simulink model "FlashMemory"  (R2016b)
settings: Solver=FixedStepAuto  StartTime=0.0  StopTime=10.0  RelTol=1e-3
PreLoadFcn:
  | waijung.modelPreload; % Required for working with Waijung Blockset. Do not remove.
undefined symbols (not defined in the file): CPHA_1Edge, CPOL_Low, deg_, Duplex, FirstBit_MSB, Full, g, imu, Link, LQFP100, ST, STM32F407VG, STM32F4DISCOVERY, Ts
libraries: simulink x45, stm32f4_i2c_lib x12, stm32f4_spi_lib x4, stm32f4_flash_lib x3, stm32f4_io_lib x1, cube_lib x1, stm32f4_device_config_lib x1, BC_USB x1
(part 1 of 3)
CloseFcn:
  | waijung.modelClose; % Required for working with Waijung Blockset. Do not remove.
settings Model: Creator=Wall  LastModifiedBy=Wall
settings OptimizationCC: DefaultParameterBehavior=Inlined
settings DebuggingCC: ParameterTunabilityLossMsg=error
settings HardwareCC: ProdBitPerPointer=32  ProdBitPerSizeT=32  ProdBitPerPtrDiffT=32  ProdLargestAtomicFloat=None  ProdIntDivRoundTo=Undefined  ProdWordSize=32  ProdHWDeviceType=ARM Compatible->Cortex - M4  TargetEndianess=LittleEndian  TargetHWDeviceType=ARM Compatible->Cortex - M4
settings RTWCC: SystemTargetFile=stm32f4.tlc  GenerateMakefile=off  TemplateMakefile=ert_default_tmf  Description=STM32F4 Target  GenerateReport=on  IncludeHyperlinkInReport=on  GenerateTraceInfo=on  GenerateTraceReport=on  GenerateTraceReportSl=on  GenerateTraceReportSf=on  GenerateTraceReportEml=on
settings CodeAppCC: ForceParamTrailComments=on  IgnoreCustomStorageClasses=off  OperatorAnnotations=on  SimulinkDataObjDesc=on  SFDataObjDesc=on  MATLABFcnDesc=on  InsertBlockDesc=on  MATLABSourceComments=on
settings STFCustomTargetCC: TargetLangStandard=C99 (ISO)  ModelReferenceCompliant=off  CombineOutputUpdateFcns=on  ERTCustomFileBanners=on  SupportContinuousTime=off  SupportNonInlinedSFcns=off  RemoveResetFunc=on  MATLABClassNameForMDSCustomization=Simulink.SoftwareTarget.ERTCustomization  GRTInterface=off  SystemTargetFile=stm32f4.tlc
settings ERTTargetCC: TargetLangStandard=C99 (ISO)  ModelReferenceCompliant=off  ParMdlRefBuildCompliant=off  CompOptLevelCompliant=off  ConcurrentExecutionCompliant=off  ERTFirstTimeCompliant=off  ModelStepFunctionPrototypeControlCompliant=off  CPPClassGenCompliant=off  UseToolchainInfoCompliant=off  InlinedParameterPlacement=NonHierarchical  ERTSrcFileBannerTemplate=stm32f4_code_template.cgt  ERTHdrFileBannerTemplate=stm32f4_code_template.cgt  ERTDataSrcFileTemplate=stm32f4_code_template.cgt  ERTDataHdrFileTemplate=stm32f4_code_template.cgt  ERTCustomFileTemplate=stm32f4_file_process.tlc

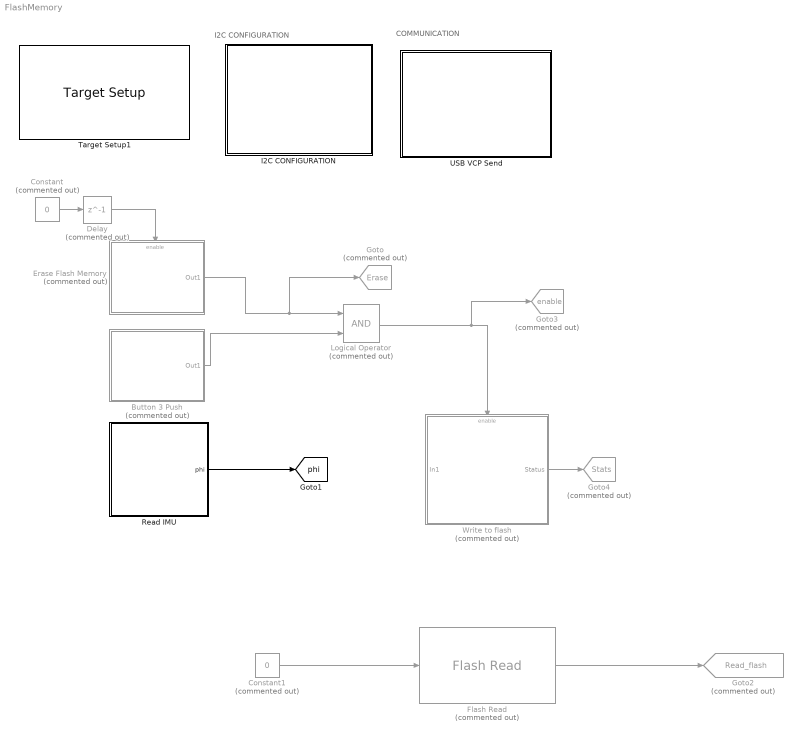
== system FlashMemory ==
  note: COMMUNICATION
  note: I2C CONFIGURATION
  Button 3 Push : Subsystem  Commented=on
  Constant : Constant  Commented=on  Value=0  SampleTime=Ts.IMU
  Constant1 : Constant  Commented=on  Value=0  OutDataTypeStr=uint32  SampleTime=-1
  Delay : Delay  Commented=on  DelayLength=1  InitialCondition=1
  Erase Flash Memory : Subsystem  Commented=on
  Flash Read : stm32f4_flash_lib/Flash Read  Commented=on  conf=Read  transfer=Blocking  flashsector=Sector 6: 0x08040000 - 0x0805FFFF  datatype=single  datacount=1  enablestatus=on  sampletime=Ts.IMU  sampletimestr=0.008  blockid=FlashRead  inputarray=[-1]  inputlabelarray={'Offset '}  outputarray=[1]  outputlabelarray={'Data (single)'}  compat=0  confstr="[\"single\",\"20000\",\"08040000\",\"6\",\"on\"]"
  Goto : Goto  Commented=on  GotoTag=Erase  TagVisibility=global
  Goto2 : Goto  Commented=on  GotoTag=Read_flash  TagVisibility=global
  Goto3 : Goto  Commented=on  GotoTag=enable  TagVisibility=global
  Goto4 : Goto  Commented=on  GotoTag=Stats  TagVisibility=global
  I2C CONFIGURATION : Subsystem
  Logical Operator : Logic  Commented=on  AllPortsSameDT=off  OutDataTypeStr=boolean
  Read IMU : Subsystem
  Target Setup1 : stm32f4_device_config_lib/Target Setup  Priority=100  compiler=GNU ARM  previous_compiler=GNU ARM  mcu=STM32F407VG (LQFP100); STM32F4DISCOVERY  mcustr=STM32F407VG  clockconfig=STM32F4DISCOVERY Default (HSEOSC-8MHz/HCLK-168MHz)  system_stm32f4xx_c_path=C:\waijung15_04a\targets\stm32f4_target\stm32f4\utils\STM32F4xx_AN3988_V1.0.1\stm32f4_default\hseosc8mhz  showmemoryconfiguration=off  stacksize=0x400  heapsize=0x200  enableautocompiledownload=on  fullchiperase=off  programmerinterface=ST-Link  editctrlstr=on  compilercontrolstr=$(patsubst %, -I%, .) -mcpu=cortex-m4 -mthumb -mthumb-interwork -mfloat-abi=hard -mfpu=fpv4-sp-d16 -ffast-math -Wall -Wextra -Ofast  assemblercontrolstr=$(patsubst %, -I%, .) -mcpu=cortex-m4 -mthumb -mthumb-interwork -mfloat-abi=hard -mfpu=fpv4-sp-d16 -ffast-math -Wall -Wextra -Ofast -Wa,-amhls=$(<:.s=.lst) -D__STACK_SIZE=$(STACK_SIZE) -D__HEAP_SIZE=$(HEAP_SIZE)  linkercontrolstr=-T$(LD_SCRIPT) -g -Wl,-Map=$(MAP),--cref,--no-warn-mismatch -mcpu=cortex-m4 -mthumb -mthumb-interwork -mfloat-abi=hard -mfpu=fpv4-sp-d16  runafterdownload=on  execprofile=None  profileruart=1  profilerbaud=115200  profilertxpin=Not used  profilerinitstr=0.002,168000000,336000,115200,0  manualsetsampletime=on  sampletime=0.002  blockid=TargetSetup1  systickreloadvalue=336000  hseval=8000000  lastprofileruart=1  hclk=168000000  flashorigin=0x8000000  flashlength=1M  ramorigin=0x20000000  ramlength=112k  useextram=off
  USB VCP Send : Subsystem
  Write to flash : Subsystem  Commented=on
  tag scope: phi=global
  wires:
  Constant/1 -> Delay/1
  Delay/1 -> Erase Flash Memory/Enable
  Erase Flash Memory/1(Out1) -> Goto/1, Logical Operator/1
  Logical Operator/1 -> Goto3/1, Write to flash/Enable
  Button 3 Push/1(Out1) -> Logical Operator/2
  Read IMU/1(phi) -> [phi]
  Constant1/1 -> Flash Read/1
  Write to flash/1(Status) -> Goto4/1
  Flash Read/1 -> Goto2/1

== system FlashMemory/Button 3 Push ==
  Buttom 3 : stm32f4_io_lib/Digital Input  port=E  speed=100  porttype=Pull Up  porttypestr=UP  use_pin0=off  use_pin1=off  use_pin2=off  use_pin3=off  use_pin4=off  use_pin5=off  use_pin6=off  use_pin7=off  use_pin8=off  use_pin9=off  use_pin10=on  use_pin11=off  use_pin12=off  use_pin13=off  use_pin14=off  use_pin15=off  pinstr=GPIO_Pin_10  usedpinarray="[0  0  0  0  0  0  0  0  0  0  1  0  0  0  0  0]"  bitbandingstr="#define Button3PushButtom3_E10 Peripheral_BB(GPIOE->IDR, 10)  /* Output pin */"  sampletime=Ts.IMU  sampletimestr=0.008  blockid=Button3PushButtom3  enablecustomportlabel=off  glabalinit=off  cinputportlabel=In1, In2  coutputportlabel=Out1, Out2
  Compare To Constant1 : simulink/Logic and Bit Operations/Compare To Constant  relop===  const=0  OutDataTypeStr=boolean  ZeroCross=off
  Rising edge boolean : cube_lib/Rising edge boolean
  Out1 : Outport
  wires:
  Rising edge boolean/1 -> Out1/1
  Buttom 3/1 -> Compare To Constant1/1
  Compare To Constant1/1 -> Rising edge boolean/1

== system FlashMemory/Erase Flash Memory ==
  Enable : EnablePort
  Compare To Zero : simulink/Logic and Bit Operations/Compare To Zero  relop===  OutDataTypeStr=boolean
  Flash Erase : stm32f4_flash_lib/Flash Erase  conf=Erase  transfer=Blocking  flashsector=Sector 6: 0x08040000 - 0x0805FFFF  datatype=uint32  datacount=1  enablestatus=on  sampletime=-1  sampletimestr=0.008  blockid=EraseFlashMemoryFlashErase  inputarray=[]  inputlabelarray={}  outputarray=[3]  outputlabelarray={'Status'}  compat=0  confstr="[\"Blocking\",\"on\",\"08040000\",\"6\"]"
  Out1 : Outport
  wires:
  Flash Erase/1 -> Compare To Zero/1
  Compare To Zero/1 -> Out1/1

== system FlashMemory/I2C CONFIGURATION ==
  I2C Master Setup1 : S-Function  FunctionName=stm32f4_i2c  Parameters=configuration,module,transfer,clkspeed,timeout,sdapin,sclpin,writecount,readcount,inputtypearray,outputtypearray,confstr,sampletime,sampletimestr,blockid  SFunctionDeploymentMode=off  EnableBusSupport=off  mask(stm32f4_i2c){configuration=Setup, module=3, lastmodule=3, transfer=Blocking, dutycycle=TLow/THigh = 2, clkspeed=400, timeout=25, writecount=0, readcount=0, sdapin=C9, sclpin=A8, waitwritetime=0, inputtypearray=[0], outputtypearray=[0], confstr=["C","9","A","8","1","3","4","2","I2C_DutyCycle_2","0","off"], sampletime=-1, sampletimestr=0.002, blockid=I2CCONFIGURATIONI2CMasterSetup1}
      mask prompts: module "I2C Module"; lastmodule "Last module"; transfer "Transfer mode"; dutycycle "Duty cycle in fast mode"; clkspeed "Clock speed (kHz)"; timeout "Timeout (ms)"; writecount "Bytes write count"; readcount "Bytes read count"; sdapin "SDA pin"; sclpin "SCL pin"; waitwritetime "Wait write time (ms), default is 0"; inputtypearray "Input type array"; outputtypearray "Output type array"; confstr "Configuration string"; sampletime "Sample time (sec)"; sampletimestr "Compiled sample time (sec) in string"
      mask init:
      | stm32f4_i2c_callback('init');
      mask Help: web(fullfile(waijungdocroot,'stm32f4_i2c_setup.htm'), '-browser')
      mask TypeOptions configuration: Setup | Transaction
      mask Callback configuration: stm32f4_i2c_callback('configuration');
      mask TypeOptions module: 1 | 2 | 3
      mask Callback module: stm32f4_i2c_callback('module');
      mask TypeOptions transfer: Blocking | Non-blocking
      mask TypeOptions dutycycle: TLow/THigh = 16/9 | TLow/THigh = 2
      mask Callback dutycycle: stm32f4_i2c_callback('dutycycle');
      mask Callback writecount: stm32f4_i2c_callback('writecount');
      mask Callback readcount: stm32f4_i2c_callback('readcount');
      mask TypeOptions sdapin: - | C9
      mask Callback sdapin: stm32f4_i2c_callback('sdapin');
      mask TypeOptions sclpin: - | A8
      mask Callback sclpin: stm32f4_i2c_callback('sclpin');
      mask Callback confstr: stm32f4_i2c_callback('confstr');
      mask Callback sampletime: stm32f4_i2c_callback('sampletime');
      mask Callback sampletimestr: stm32f4_i2c_callback('sampletimestr');
      mask Callback blockid: stm32f4_i2c_callback('blockid');
      mask Display: text(0.5, 0.5, 'Module: I2C3\nClock: 400kHz\nSDA/SCL Pin: C9/A8','ver','middle','hor','center');
  I2C Master Setup2 : S-Function  FunctionName=stm32f4_i2c  Parameters=configuration,module,transfer,clkspeed,timeout,sdapin,sclpin,writecount,readcount,inputtypearray,outputtypearray,confstr,sampletime,sampletimestr,blockid  SFunctionDeploymentMode=off  EnableBusSupport=off  mask(stm32f4_i2c){configuration=Setup, module=1, lastmodule=1, transfer=Blocking, dutycycle=TLow/THigh = 2, clkspeed=400, timeout=25, writecount=0, readcount=0, sdapin=B9, sclpin=B6, waitwritetime=0, inputtypearray=[0], outputtypearray=[0], confstr=["B","9","B","6","1","1","6","0","I2C_DutyCycle_2","0","off"], sampletime=-1, sampletimestr=0.002, blockid=I2CCONFIGURATIONI2CMasterSetup2}
      mask prompts: module "I2C Module"; lastmodule "Last module"; transfer "Transfer mode"; dutycycle "Duty cycle in fast mode"; clkspeed "Clock speed (kHz)"; timeout "Timeout (ms)"; writecount "Bytes write count"; readcount "Bytes read count"; sdapin "SDA pin"; sclpin "SCL pin"; waitwritetime "Wait write time (ms), default is 0"; inputtypearray "Input type array"; outputtypearray "Output type array"; confstr "Configuration string"; sampletime "Sample time (sec)"; sampletimestr "Compiled sample time (sec) in string"
      mask init:
      | stm32f4_i2c_callback('init');
      mask Help: web(fullfile(waijungdocroot,'stm32f4_i2c_setup.htm'), '-browser')
      mask TypeOptions configuration: Setup | Transaction
      mask Callback configuration: stm32f4_i2c_callback('configuration');
      mask TypeOptions module: 1 | 2 | 3
      mask Callback module: stm32f4_i2c_callback('module');
      mask TypeOptions transfer: Blocking | Non-blocking
      mask TypeOptions dutycycle: TLow/THigh = 16/9 | TLow/THigh = 2
      mask Callback dutycycle: stm32f4_i2c_callback('dutycycle');
      mask Callback writecount: stm32f4_i2c_callback('writecount');
      mask Callback readcount: stm32f4_i2c_callback('readcount');
      mask TypeOptions sdapin: - | B7 | B9
      mask Callback sdapin: stm32f4_i2c_callback('sdapin');
      mask TypeOptions sclpin: - | B6 | B8
      mask Callback sclpin: stm32f4_i2c_callback('sclpin');
      mask Callback confstr: stm32f4_i2c_callback('confstr');
      mask Callback sampletime: stm32f4_i2c_callback('sampletime');
      mask Callback sampletimestr: stm32f4_i2c_callback('sampletimestr');
      mask Callback blockid: stm32f4_i2c_callback('blockid');
      mask Display: text(0.5, 0.5, 'Module: I2C1\nClock: 400kHz\nSDA/SCL Pin: B9/B6','ver','middle','hor','center');

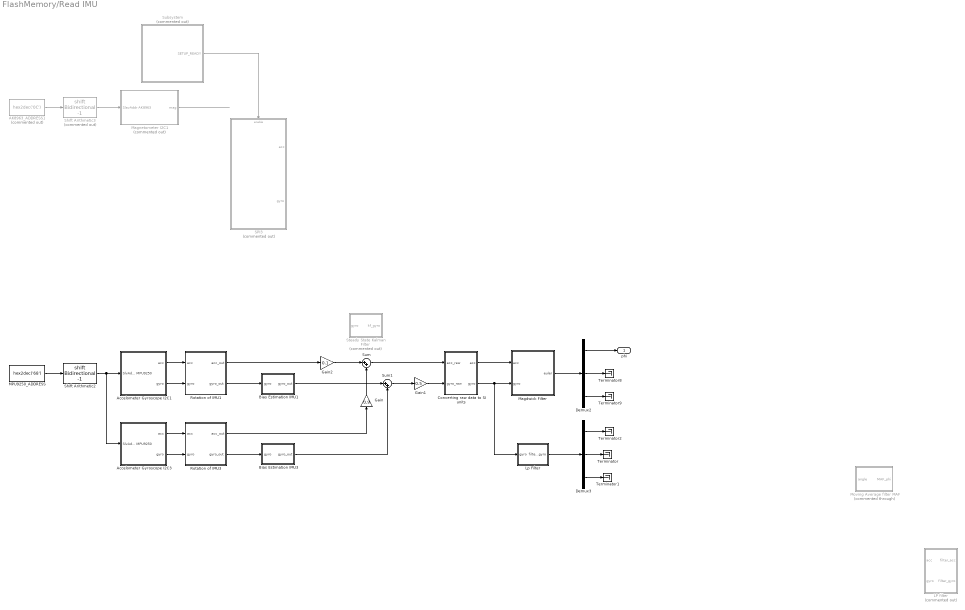
== system FlashMemory/Read IMU ==
  " AK8963_ADDRESS1" : Constant  Commented=on  Value=hex2dec('0C')  OutDataTypeStr=uint8  SampleTime=0.002
  " MPU9250_ADDRESS" : Constant  Value=hex2dec('68')  OutDataTypeStr=uint8  SampleTime=Ts.IMU
  Accelometer Gyroscope I2C1 : Subsystem
  Accelometer Gyroscope I2C3 : Subsystem
  Bias Estimation IMU1 : MATLAB Function  TreatAsAtomicUnit=on
  Bias Estimation IMU3 : MATLAB Function  TreatAsAtomicUnit=on
  Converting raw data to SI units : Subsystem
  Demux2 : Demux  Outputs=3
  Demux3 : Demux  Outputs=3
  Gain : Gain  Gain=0.9
  Gain1 : Gain  Gain=0.5
  Gain2 : Gain  Gain=0.1
  LP filter : MATLAB Function  Commented=on  TreatAsAtomicUnit=on
  Lp Filter : MATLAB Function  TreatAsAtomicUnit=on
  Magdwick Filter : MATLAB Function  TreatAsAtomicUnit=on
  Magnetometer I2C1 : Subsystem  Commented=on
  Moving Average filter MAF : MATLAB Function  Commented=through  TreatAsAtomicUnit=on
  Rotation of IMU1 : MATLAB Function  TreatAsAtomicUnit=on
  Rotation of IMU3 : MATLAB Function  TreatAsAtomicUnit=on
  SPI3 : Subsystem  Commented=on
  Shift Arithmetic2 : ArithShift  BitShiftNumber=-1
  Shift Arithmetic3 : ArithShift  Commented=on  BitShiftNumber=-1
  Steady State Kalman Filter : MATLAB Function  Commented=on  TreatAsAtomicUnit=on
  Subsystem : Subsystem  Commented=on
  Sum : Sum  Inputs=|++
  Sum1 : Sum  Inputs=|++
  Terminator{,1..2,8..9} (5 alike) : Terminator
  phi : Outport
  wires:
  Demux3/2 -> Terminator/1
  Demux2/2 -> Terminator8/1
  Demux2/3 -> Terminator9/1
  Demux3/3 -> Terminator1/1
  Converting raw data to SI units/1(acc) -> Magdwick Filter/1(acc)
  Demux3/1 -> Terminator2/1
  Lp Filter/1(filter_gyro) -> Demux3/1
  Magdwick Filter/1(euler) -> Demux2/1
  Converting raw data to SI units/2(gyro) -> Magdwick Filter/2(gyro), Lp Filter/1(gyro)
  Accelometer Gyroscope I2C1/2(gyro) -> Rotation of IMU1/2(gyro)
  Subsystem/1(SETUP_READY) -> SPI3/Enable
  Shift Arithmetic2/1 -> Accelometer Gyroscope I2C3/1(SlvAddr MPU9250), Accelometer Gyroscope I2C1/1(SlvAddr MPU9250)
  Accelometer Gyroscope I2C1/1(acc) -> Rotation of IMU1/1(acc)
  " MPU9250_ADDRESS"/1 -> Shift Arithmetic2/1
  Shift Arithmetic3/1 -> Magnetometer I2C1/1(SlavAddr AK8963)
  " AK8963_ADDRESS1"/1 -> Shift Arithmetic3/1
  Magnetometer I2C1/1(mag) -> ?
  Accelometer Gyroscope I2C3/1(acc) -> Rotation of IMU3/1(acc)
  Accelometer Gyroscope I2C3/2(gyro) -> Rotation of IMU3/2(gyro)
  Rotation of IMU1/2(gyro_out) -> Bias Estimation IMU1/1(gyro)
  Rotation of IMU3/2(gyro_out) -> Bias Estimation IMU3/1(gyro)
  Sum1/1 -> Gain1/1
  Sum/1 -> Converting raw data to SI units/1(acc_raw)
  Bias Estimation IMU1/1(gyro_out) -> Sum1/1
  Gain2/1 -> Sum/1
  Gain/1 -> Sum/2
  Gain1/1 -> Converting raw data to SI units/2(gyro_raw)
  Bias Estimation IMU3/1(gyro_out) -> Sum1/2
  Rotation of IMU3/1(acc_out) -> Gain/1
  Rotation of IMU1/1(acc_out) -> Gain2/1
  Demux2/1 -> phi/1

== system FlashMemory/USB VCP Send ==
  Data Type Conversion{,1..3} (4 alike) : DataTypeConversion
  USB VCP Send STM32F1 : BC_USB/USB VCP Send STM32F4  speed="USB 1.1   12Mbit/s"  data_size=2048 Bytes  header_data='0E 0E'  binary_data='single single single single'  terminator_data='0A 0A'  sampletime=Ts.base
  wires:
  [phi] -> Data Type Conversion/1
  Data Type Conversion/1 -> USB VCP Send STM32F1/1
  [Stats] -> Data Type Conversion1/1
  Data Type Conversion1/1 -> USB VCP Send STM32F1/2
  [Erase] -> Data Type Conversion2/1
  Data Type Conversion2/1 -> USB VCP Send STM32F1/3
  [Read_flash] -> Data Type Conversion3/1
  Data Type Conversion3/1 -> USB VCP Send STM32F1/4

== system FlashMemory/Write to flash ==
  In1 : Inport
  Enable : EnablePort
  Compare To Zero : simulink/Logic and Bit Operations/Compare To Zero  relop===  OutDataTypeStr=boolean
  Constant : Constant  Value=0  OutDataTypeStr=uint32  SampleTime=-1
  Flash Write : stm32f4_flash_lib/Flash Write  conf=Program  transfer=Blocking  flashsector=Sector 6: 0x08040000 - 0x0805FFFF  datatype=single  datacount=1  enablestatus=on  sampletime=-1  sampletimestr=0.002  blockid=WritetoflashFlashWrite  inputarray=[-1,1]  inputlabelarray={'Offset ', 'Data (single)'}  outputarray=[3]  outputlabelarray={'Status'}  compat=0  confstr="[\"Blocking\",\"single\",\"on\",\"20000\",\"08040000\",\"6\"]"
  Status : Outport
  wires:
  Constant/1 -> Flash Write/1
  Flash Write/1 -> Compare To Zero/1
  Compare To Zero/1 -> Status/1
  In1/1 -> Flash Write/2

== system FlashMemory/Read IMU/Accelometer Gyroscope I2C1 ==
  SlvAddr MPU9250 : Inport
  MPU9250 Init : Subsystem
  Read Accelometer and Gyroscope Data : Subsystem
  acc : Outport
  gyro : Outport  Port=2
  wires:
  SlvAddr MPU9250/1 -> Read Accelometer and Gyroscope Data/1(SlvAddr), MPU9250 Init/1(SlvAddr)
  Read Accelometer and Gyroscope Data/1(acc) -> acc/1
  Read Accelometer and Gyroscope Data/2(gyro) -> gyro/1
  MPU9250 Init/1(SETUP_READY) -> Read Accelometer and Gyroscope Data/Enable

== system FlashMemory/Read IMU/Accelometer Gyroscope I2C3 ==
  SlvAddr MPU9250 : Inport
  MPU9250 Init : Subsystem
  Read Accelometer and Gyroscope Data : Subsystem
  acc : Outport
  gyro : Outport  Port=2
  wires:
  SlvAddr MPU9250/1 -> Read Accelometer and Gyroscope Data/1(SlvAddr), MPU9250 Init/1(SlvAddr)
  Read Accelometer and Gyroscope Data/1(acc) -> acc/1
  Read Accelometer and Gyroscope Data/2(gyro) -> gyro/1
  MPU9250 Init/1(SETUP_READY) -> Read Accelometer and Gyroscope Data/Enable

== system FlashMemory/Read IMU/Converting raw data to SI units ==
  acc_raw : Inport
  gyro_raw : Inport  Port=2
  Raw sensor value to SI units Accelometer : Gain  Gain=1 / imu.a_scaling * g
  Raw sensor value to SI units Gyroscope : Gain  Gain=1 / imu.w_scaling * deg_
  acc : Outport
  gyro : Outport  Port=2
  wires:
  gyro_raw/1 -> Raw sensor value to SI units Gyroscope/1
  Raw sensor value to SI units Accelometer/1 -> acc/1
  Raw sensor value to SI units Gyroscope/1 -> gyro/1
  acc_raw/1 -> Raw sensor value to SI units Accelometer/1

== system FlashMemory/Read IMU/Magnetometer I2C1 ==
  note: Read magnetometer data for the third party sensor on the MPU9250
  SlavAddr AK8963 : Inport
  "AK8963 Init " : Subsystem
  "Magnetometer Data Ready " : Subsystem
  Read Magnetometer Data : Subsystem
  mag : Outport
  wires:
  "AK8963 Init "/1(READY) -> "Magnetometer Data Ready "/Enable
  Read Magnetometer Data/1(mag) -> mag/1
  SlavAddr AK8963/1 -> "Magnetometer Data Ready "/1(SlvAddr), Read Magnetometer Data/1("SlvAddr "), "AK8963 Init "/1(SlvAddr)
  "Magnetometer Data Ready "/1(READY) -> Read Magnetometer Data/Enable

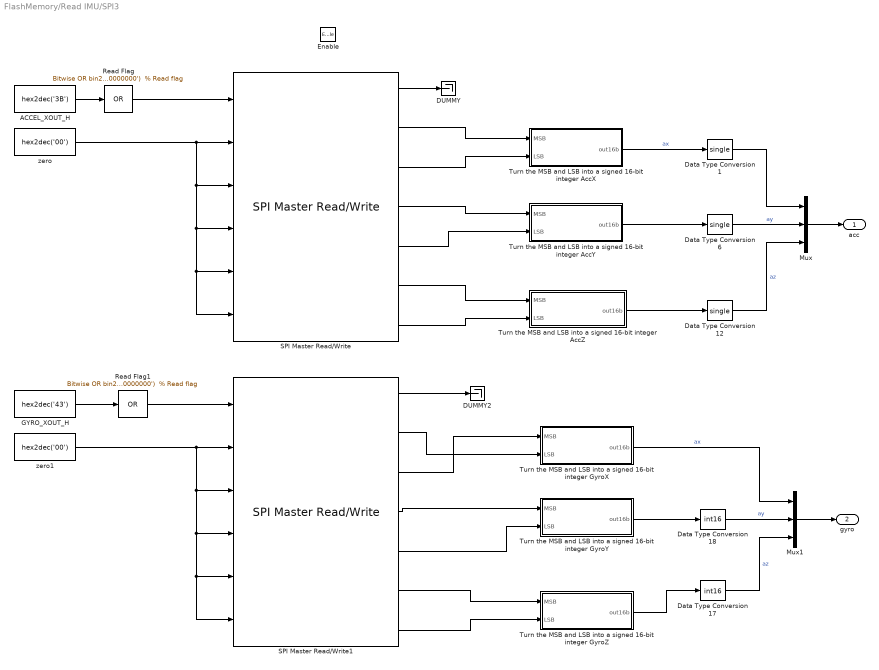
== system FlashMemory/Read IMU/SPI3 ==
  Enable : EnablePort
  ACCEL_XOUT_H : Constant  Value=hex2dec('3B')  OutDataTypeStr=uint8  SampleTime=-1
  DUMMY : Terminator
  DUMMY2 : Terminator
  Data Type Conversion1 : DataTypeConversion  OutDataTypeStr=single
  Data Type Conversion12 : DataTypeConversion  OutDataTypeStr=single
  Data Type Conversion17 : DataTypeConversion  OutDataTypeStr=int16
  Data Type Conversion18 : DataTypeConversion  OutDataTypeStr=int16
  Data Type Conversion6 : DataTypeConversion  OutDataTypeStr=single
  GYRO_XOUT_H : Constant  Value=hex2dec('43')  OutDataTypeStr=uint8  SampleTime=-1
  Mux : Mux  Inputs=3
  Mux1 : Mux  Inputs=3
  Read Flag : simulink/Logic and Bit Operations/Bitwise Operator  logicop=OR  UseBitMask=on  BitMask="bin2dec('10000000')  % Read flag"  BitMaskRealWorld=Real World Value
  Read Flag1 : simulink/Logic and Bit Operations/Bitwise Operator  logicop=OR  UseBitMask=on  BitMask="bin2dec('10000000')  % Read flag"  BitMaskRealWorld=Real World Value
  SPI Master Read/Write : stm32f4_spi_lib/SPI Master Read//Write  configuration=Transaction  module=3  mode=Read/ Write  lastmodule=1  direction=Full-Duplex  dataformat=8bit/ FirstBit_MSB  prescaler=4  cpolcpha=CPOL_Low/ CPHA_1Edge  datacount=6  nssmode=Custom  nsspin=Not used  softnssport=E  softnsspin=0  sckpin=A5  misopin=A6  mosipin=A7  inputtypearray=[6 3 3 3 3 3 3]  outputtypearray=[7 7 3 3 3 3 3 3]  confstr="[\"SPI_Direction_2Lines_FullDuplex\",\"8b\",\"MSB\",\"Low\",\"1Edge\",\"4\",\"Soft\",\"0\",\"x\",\"x\",\"0\",\"x\",\"x\",\"1\",\"A\",\"5\",\"1\",\"A\",\"6\",\"1\",\"A\",\"7\",\"1\",\"0\",\"0\",\"0\",\"0\",\"0\",\"0\",\"0\",\"0\",\"PP\",\"0\",\"UP\"]"  sampletime=0.002  sampletimestr=0.002  blockid=ReadIMUSPI3SPIMasterReadWrite
  SPI Master Read/Write1 : stm32f4_spi_lib/SPI Master Read//Write  configuration=Transaction  module=3  mode=Read/ Write  lastmodule=1  direction=Full-Duplex  dataformat=8bit/ FirstBit_MSB  prescaler=4  cpolcpha=CPOL_Low/ CPHA_1Edge  datacount=6  nssmode=Custom  nsspin=Not used  softnssport=E  softnsspin=0  sckpin=A5  misopin=A6  mosipin=A7  inputtypearray=[6 3 3 3 3 3 3]  outputtypearray=[7 7 3 3 3 3 3 3]  confstr="[\"SPI_Direction_2Lines_FullDuplex\",\"8b\",\"MSB\",\"Low\",\"1Edge\",\"4\",\"Soft\",\"0\",\"x\",\"x\",\"0\",\"x\",\"x\",\"1\",\"A\",\"5\",\"1\",\"A\",\"6\",\"1\",\"A\",\"7\",\"1\",\"0\",\"0\",\"0\",\"0\",\"0\",\"0\",\"0\",\"0\",\"PP\",\"0\",\"UP\"]"  sampletime=0.002  sampletimestr=0.002  blockid=ReadIMUSPI3SPIMasterReadWrite1
  Turn the MSB and LSB into a signed 16-bit integer AccX : Subsystem
  Turn the MSB and LSB into a signed 16-bit integer AccY : Subsystem
  Turn the MSB and LSB into a signed 16-bit integer AccZ : Subsystem
  Turn the MSB and LSB into a signed 16-bit integer GyroX : Subsystem
  Turn the MSB and LSB into a signed 16-bit integer GyroY : Subsystem
  Turn the MSB and LSB into a signed 16-bit integer GyroZ : Subsystem
  zero : Constant  Value=hex2dec('00')  OutDataTypeStr=uint8  SampleTime=-1
  zero1 : Constant  Value=hex2dec('00')  OutDataTypeStr=uint8  SampleTime=-1
  acc : Outport
  gyro : Outport  Port=2
  wires:
  Data Type Conversion6/1 -> Mux/2  "ay"
  Mux1/1 -> gyro/1
  GYRO_XOUT_H/1 -> Read Flag1/1
  SPI Master Read/Write/1 -> DUMMY/1
  SPI Master Read/Write1/1 -> DUMMY2/1
  Mux/1 -> acc/1
  Data Type Conversion18/1 -> Mux1/2  "ay"
  Turn the MSB and LSB into a signed 16-bit integer GyroZ/1(out16b) -> Data Type Conversion17/1
  Turn the MSB and LSB into a signed 16-bit integer AccX/1(out16b) -> Data Type Conversion1/1  "ax"
  Turn the MSB and LSB into a signed 16-bit integer GyroY/1(out16b) -> Data Type Conversion18/1
  Turn the MSB and LSB into a signed 16-bit integer GyroX/1(out16b) -> Mux1/1  "ax"
  Turn the MSB and LSB into a signed 16-bit integer AccY/1(out16b) -> Data Type Conversion6/1
  Turn the MSB and LSB into a signed 16-bit integer AccZ/1(out16b) -> Data Type Conversion12/1
  Data Type Conversion12/1 -> Mux/3  "az"
  Data Type Conversion17/1 -> Mux1/3  "az"
  ACCEL_XOUT_H/1 -> Read Flag/1
  Read Flag/1 -> SPI Master Read/Write/1
  zero/1 -> SPI Master Read/Write/6, SPI Master Read/Write/5, SPI Master Read/Write/4, SPI Master Read/Write/3, SPI Master Read/Write/2
  Read Flag1/1 -> SPI Master Read/Write1/1
  zero1/1 -> SPI Master Read/Write1/6, SPI Master Read/Write1/5, SPI Master Read/Write1/4, SPI Master Read/Write1/3, SPI Master Read/Write1/2
  SPI Master Read/Write1/4 -> Turn the MSB and LSB into a signed 16-bit integer GyroY/1(MSB)
  SPI Master Read/Write1/5 -> Turn the MSB and LSB into a signed 16-bit integer GyroY/2(LSB)
  SPI Master Read/Write1/6 -> Turn the MSB and LSB into a signed 16-bit integer GyroZ/1(MSB)
  SPI Master Read/Write1/7 -> Turn the MSB and LSB into a signed 16-bit integer GyroZ/2(LSB)
  SPI Master Read/Write/2 -> Turn the MSB and LSB into a signed 16-bit integer AccX/1(MSB)
  SPI Master Read/Write/3 -> Turn the MSB and LSB into a signed 16-bit integer AccX/2(LSB)
  SPI Master Read/Write/4 -> Turn the MSB and LSB into a signed 16-bit integer AccY/1(MSB)
  SPI Master Read/Write/5 -> Turn the MSB and LSB into a signed 16-bit integer AccY/2(LSB)
  SPI Master Read/Write/6 -> Turn the MSB and LSB into a signed 16-bit integer AccZ/1(MSB)
  SPI Master Read/Write/7 -> Turn the MSB and LSB into a signed 16-bit integer AccZ/2(LSB)
  Data Type Conversion1/1 -> Mux/1
  SPI Master Read/Write1/3 -> Turn the MSB and LSB into a signed 16-bit integer GyroX/1(MSB)
  SPI Master Read/Write1/2 -> Turn the MSB and LSB into a signed 16-bit integer GyroX/2(LSB)

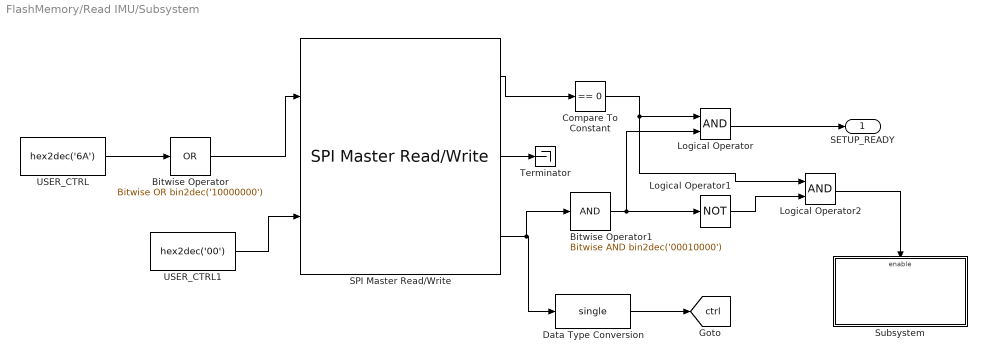
== system FlashMemory/Read IMU/Subsystem ==
  Bitwise Operator : simulink/Logic and Bit Operations/Bitwise Operator  logicop=OR  UseBitMask=on  BitMask=bin2dec('10000000')  BitMaskRealWorld=Stored Integer
  Bitwise Operator1 : simulink/Logic and Bit Operations/Bitwise Operator  logicop=AND  UseBitMask=on  BitMask=bin2dec('00010000')  BitMaskRealWorld=Stored Integer
  Compare To Constant : simulink/Logic and Bit Operations/Compare To Constant  relop===  const=0  OutDataTypeStr=boolean
  Data Type Conversion : DataTypeConversion  OutDataTypeStr=single
  Logical Operator : Logic  AllPortsSameDT=off  OutDataTypeStr=boolean
  Logical Operator1 : Logic  Operator=NOT  AllPortsSameDT=off  OutDataTypeStr=boolean
  Logical Operator2 : Logic  AllPortsSameDT=off  OutDataTypeStr=boolean
  SPI Master Read/Write : stm32f4_spi_lib/SPI Master Read//Write  configuration=Transaction  module=3  mode=Read/ Write  lastmodule=1  direction=Full-Duplex  dataformat=8bit/ FirstBit_MSB  prescaler=4  cpolcpha=CPOL_Low/ CPHA_1Edge  datacount=2  nssmode=Custom  nsspin=Not used  softnssport=E  softnsspin=0  sckpin=A5  misopin=A6  mosipin=A7  inputtypearray=[2 3 3]  outputtypearray=[3 7 3 3]  confstr="[\"SPI_Direction_2Lines_FullDuplex\",\"8b\",\"MSB\",\"Low\",\"1Edge\",\"4\",\"Soft\",\"0\",\"x\",\"x\",\"0\",\"x\",\"x\",\"1\",\"A\",\"5\",\"1\",\"A\",\"6\",\"1\",\"A\",\"7\",\"1\",\"0\",\"0\",\"0\",\"0\",\"0\",\"0\",\"0\",\"0\",\"PP\",\"0\",\"UP\"]"  sampletime=0.002  sampletimestr=0.002  blockid=ReadIMUSubsystemSPIMasterReadWrite
  Subsystem : Subsystem
  Terminator : Terminator
  USER_CTRL : Constant  Value=hex2dec('6A')  OutDataTypeStr=uint8  SampleTime=-1
  USER_CTRL1 : Constant  Value=hex2dec('00')  OutDataTypeStr=uint8  SampleTime=-1
  SETUP_READY : Outport
  tag scope: ctrl=global
  wires:
  Bitwise Operator/1 -> SPI Master Read/Write/1
  USER_CTRL/1 -> Bitwise Operator/1
  SPI Master Read/Write/1 -> Compare To Constant/1
  Logical Operator/1 -> SETUP_READY/1
  Compare To Constant/1 -> Logical Operator/1, Logical Operator2/1
  Bitwise Operator1/1 -> Logical Operator/2, Logical Operator1/1
  Logical Operator1/1 -> Logical Operator2/2
  Logical Operator2/1 -> Subsystem/Enable
  Data Type Conversion/1 -> [ctrl]
  SPI Master Read/Write/3 -> Bitwise Operator1/1, Data Type Conversion/1
  USER_CTRL1/1 -> SPI Master Read/Write/2
  SPI Master Read/Write/2 -> Terminator/1

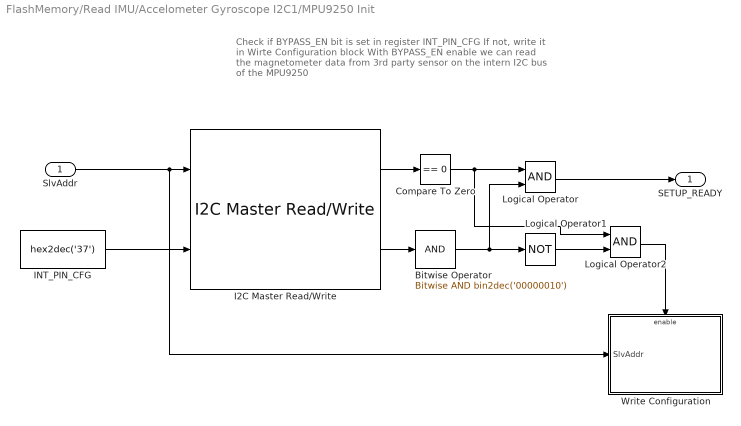
== system FlashMemory/Read IMU/Accelometer Gyroscope I2C1/MPU9250 Init ==
  note: Check if BYPASS_EN bit is set in register INT_PIN_CFG
      | If not, write it in Wirte Configuration block
      |
      | With BYPASS_EN enable we can read the magnetometer data
      | from 3rd party sensor on the intern I2C bus of the MPU9250
  SlvAddr : Inport
  Bitwise Operator : simulink/Logic and Bit Operations/Bitwise Operator  logicop=AND  UseBitMask=on  BitMask=bin2dec('00000010')  BitMaskRealWorld=Stored Integer
  Compare To Zero : simulink/Logic and Bit Operations/Compare To Zero  relop===  OutDataTypeStr=boolean
  I2C Master Read/Write : stm32f4_i2c_lib/I2C Master Read//Write  configuration=Transaction  module=1  lastmodule=3  transfer=Blocking  dutycycle=TLow/THigh = 2  clkspeed=400  timeout=25  writecount=1  readcount=1  sdapin=C9  sclpin=A8  waitwritetime=0  forcestop=off  inputtypearray=[2 3 3]  outputtypearray=[2 3 3]  confstr="[\"C\",\"9\",\"A\",\"8\",\"1\",\"1\",\"6\",\"0\",\"I2C_DutyCycle_2\",\"0\",\"off\"]"  sampletime=-1  sampletimestr=0.008  blockid=ReadIMUAccelometerGyroscopeI2C1MPU9250InitI2CMasterReadWrite
  INT_PIN_CFG : Constant  Value=hex2dec('37')  OutDataTypeStr=uint8  SampleTime=-1
  Logical Operator : Logic  AllPortsSameDT=off  OutDataTypeStr=boolean
  Logical Operator1 : Logic  Operator=NOT  AllPortsSameDT=off  OutDataTypeStr=boolean
  Logical Operator2 : Logic  AllPortsSameDT=off  OutDataTypeStr=boolean
  Write Configuration : Subsystem
  SETUP_READY : Outport
  wires:
  I2C Master Read/Write/1 -> Compare To Zero/1
  INT_PIN_CFG/1 -> I2C Master Read/Write/2
  SlvAddr/1 -> Write Configuration/1(SlvAddr), I2C Master Read/Write/1
  Logical Operator/1 -> SETUP_READY/1
  Compare To Zero/1 -> Logical Operator2/1, Logical Operator/1
  Bitwise Operator/1 -> Logical Operator1/1, Logical Operator/2
  Logical Operator1/1 -> Logical Operator2/2
  Logical Operator2/1 -> Write Configuration/Enable
  I2C Master Read/Write/2 -> Bitwise Operator/1

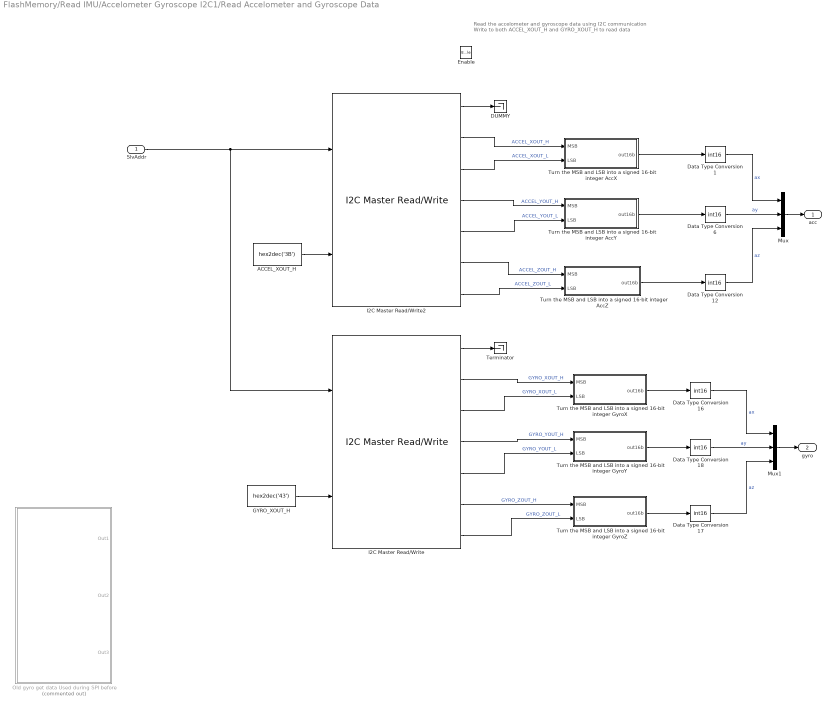
== system FlashMemory/Read IMU/Accelometer Gyroscope I2C1/Read Accelometer and Gyroscope Data ==
  note: Read the accelometer and gyroscope data using I2C communication
      | Write to both ACCEL_XOUT_H and GYRO_XOUT_H to read data
  SlvAddr : Inport
  Enable : EnablePort
  ACCEL_XOUT_H : Constant  Value=hex2dec('3B')  OutDataTypeStr=uint8  SampleTime=-1
  DUMMY : Terminator
  Data Type Conversion{1,6,12,16..18} (6 alike) : DataTypeConversion  OutDataTypeStr=int16
  GYRO_XOUT_H : Constant  Value=hex2dec('43')  OutDataTypeStr=uint8  SampleTime=-1
  I2C Master Read/Write : stm32f4_i2c_lib/I2C Master Read//Write  configuration=Transaction  module=1  lastmodule=3  transfer=Blocking  dutycycle=TLow/THigh = 2  clkspeed=400  timeout=25  writecount=1  readcount=6  sdapin=C9  sclpin=A8  waitwritetime=0  forcestop=off  inputtypearray=[2 3 3]  outputtypearray=[7 3 3 3 3 3 3 3]  confstr="[\"C\",\"9\",\"A\",\"8\",\"1\",\"1\",\"6\",\"0\",\"I2C_DutyCycle_2\",\"0\",\"off\"]"  sampletime=Ts.IMU  sampletimestr=0.008  blockid=ReadIMUAccelometerGyroscopeI2C1ReadAccelometerandGyroscopeDataI2CMasterReadWrite
  I2C Master Read/Write2 : stm32f4_i2c_lib/I2C Master Read//Write  configuration=Transaction  module=1  lastmodule=3  transfer=Blocking  dutycycle=TLow/THigh = 2  clkspeed=400  timeout=25  writecount=1  readcount=6  sdapin=C9  sclpin=A8  waitwritetime=0  forcestop=off  inputtypearray=[2 3 3]  outputtypearray=[7 3 3 3 3 3 3 3]  confstr="[\"C\",\"9\",\"A\",\"8\",\"1\",\"1\",\"6\",\"0\",\"I2C_DutyCycle_2\",\"0\",\"off\"]"  sampletime=Ts.IMU  sampletimestr=0.008  blockid=ReadIMUAccelometerGyroscopeI2C1ReadAccelometerandGyroscopeDataI2CMasterReadWrite2
  Mux : Mux  Inputs=3
  Mux1 : Mux  Inputs=3
  Old gyro get data Used during SPI before : Subsystem  Commented=on
  Terminator : Terminator
  Turn the MSB and LSB into a signed 16-bit integer AccX : Subsystem
  Turn the MSB and LSB into a signed 16-bit integer AccY : Subsystem
  Turn the MSB and LSB into a signed 16-bit integer AccZ : Subsystem
  Turn the MSB and LSB into a signed 16-bit integer GyroX : Subsystem
  Turn the MSB and LSB into a signed 16-bit integer GyroY : Subsystem
  Turn the MSB and LSB into a signed 16-bit integer GyroZ : Subsystem
  acc : Outport
  gyro : Outport  Port=2
  wires:
  I2C Master Read/Write2/1 -> DUMMY/1
  Mux/1 -> acc/1
  Turn the MSB and LSB into a signed 16-bit integer AccX/1(out16b) -> Data Type Conversion1/1
  Turn the MSB and LSB into a signed 16-bit integer AccY/1(out16b) -> Data Type Conversion6/1
  Turn the MSB and LSB into a signed 16-bit integer AccZ/1(out16b) -> Data Type Conversion12/1
  Data Type Conversion1/1 -> Mux/1  "ax"
  Data Type Conversion6/1 -> Mux/2  "ay"
  Data Type Conversion12/1 -> Mux/3  "az"
  Mux1/1 -> gyro/1
  Turn the MSB and LSB into a signed 16-bit integer GyroX/1(out16b) -> Data Type Conversion16/1
  Turn the MSB and LSB into a signed 16-bit integer GyroY/1(out16b) -> Data Type Conversion18/1
  Turn the MSB and LSB into a signed 16-bit integer GyroZ/1(out16b) -> Data Type Conversion17/1
  Data Type Conversion16/1 -> Mux1/1  "ax"
  Data Type Conversion18/1 -> Mux1/2  "ay"
  Data Type Conversion17/1 -> Mux1/3  "az"
  GYRO_XOUT_H/1 -> I2C Master Read/Write/2
  ACCEL_XOUT_H/1 -> I2C Master Read/Write2/2
  SlvAddr/1 -> I2C Master Read/Write/1, I2C Master Read/Write2/1
  I2C Master Read/Write2/2 -> Turn the MSB and LSB into a signed 16-bit integer AccX/1(MSB)  "ACCEL_XOUT_H"
  I2C Master Read/Write2/3 -> Turn the MSB and LSB into a signed 16-bit integer AccX/2(LSB)  "ACCEL_XOUT_L"
  I2C Master Read/Write2/5 -> Turn the MSB and LSB into a signed 16-bit integer AccY/2(LSB)  "ACCEL_YOUT_L"
  I2C Master Read/Write2/4 -> Turn the MSB and LSB into a signed 16-bit integer AccY/1(MSB)  "ACCEL_YOUT_H"
  I2C Master Read/Write2/6 -> Turn the MSB and LSB into a signed 16-bit integer AccZ/1(MSB)  "ACCEL_ZOUT_H"
  I2C Master Read/Write2/7 -> Turn the MSB and LSB into a signed 16-bit integer AccZ/2(LSB)  "ACCEL_ZOUT_L"
  I2C Master Read/Write/2 -> Turn the MSB and LSB into a signed 16-bit integer GyroX/1(MSB)  "GYRO_XOUT_H"
  I2C Master Read/Write/3 -> Turn the MSB and LSB into a signed 16-bit integer GyroX/2(LSB)  "GYRO_XOUT_L"
  I2C Master Read/Write/4 -> Turn the MSB and LSB into a signed 16-bit integer GyroY/1(MSB)  "GYRO_YOUT_H"
  I2C Master Read/Write/5 -> Turn the MSB and LSB into a signed 16-bit integer GyroY/2(LSB)  "GYRO_YOUT_L"
  I2C Master Read/Write/6 -> Turn the MSB and LSB into a signed 16-bit integer GyroZ/1(MSB)  "GYRO_ZOUT_H"
  I2C Master Read/Write/7 -> Turn the MSB and LSB into a signed 16-bit integer GyroZ/2(LSB)  "GYRO_ZOUT_L"
  I2C Master Read/Write/1 -> Terminator/1

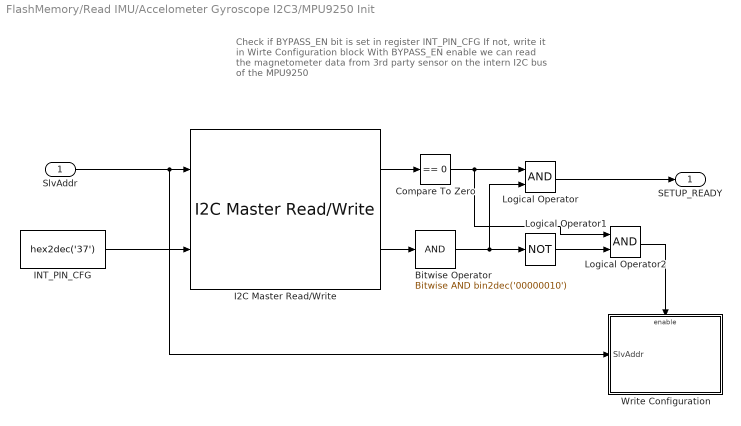
== system FlashMemory/Read IMU/Accelometer Gyroscope I2C3/MPU9250 Init ==
  note: Check if BYPASS_EN bit is set in register INT_PIN_CFG
      | If not, write it in Wirte Configuration block
      |
      | With BYPASS_EN enable we can read the magnetometer data
      | from 3rd party sensor on the intern I2C bus of the MPU9250
  SlvAddr : Inport
  Bitwise Operator : simulink/Logic and Bit Operations/Bitwise Operator  logicop=AND  UseBitMask=on  BitMask=bin2dec('00000010')  BitMaskRealWorld=Stored Integer
  Compare To Zero : simulink/Logic and Bit Operations/Compare To Zero  relop===  OutDataTypeStr=boolean
  I2C Master Read/Write : stm32f4_i2c_lib/I2C Master Read//Write  configuration=Transaction  module=3  lastmodule=3  transfer=Blocking  dutycycle=TLow/THigh = 2  clkspeed=400  timeout=25  writecount=1  readcount=1  sdapin=C9  sclpin=A8  waitwritetime=0  forcestop=off  inputtypearray=[2 3 3]  outputtypearray=[2 3 3]  confstr="[\"C\",\"9\",\"A\",\"8\",\"1\",\"3\",\"4\",\"2\",\"I2C_DutyCycle_2\",\"0\",\"off\"]"  sampletime=-1  sampletimestr=0.008  blockid=ReadIMUAccelometerGyroscopeI2C3MPU9250InitI2CMasterReadWrite
  INT_PIN_CFG : Constant  Value=hex2dec('37')  OutDataTypeStr=uint8  SampleTime=-1
  Logical Operator : Logic  AllPortsSameDT=off  OutDataTypeStr=boolean
  Logical Operator1 : Logic  Operator=NOT  AllPortsSameDT=off  OutDataTypeStr=boolean
  Logical Operator2 : Logic  AllPortsSameDT=off  OutDataTypeStr=boolean
  Write Configuration : Subsystem
  SETUP_READY : Outport
  wires:
  I2C Master Read/Write/1 -> Compare To Zero/1
  INT_PIN_CFG/1 -> I2C Master Read/Write/2
  SlvAddr/1 -> Write Configuration/1(SlvAddr), I2C Master Read/Write/1
  Logical Operator/1 -> SETUP_READY/1
  Compare To Zero/1 -> Logical Operator2/1, Logical Operator/1
  Bitwise Operator/1 -> Logical Operator1/1, Logical Operator/2
  Logical Operator1/1 -> Logical Operator2/2
  Logical Operator2/1 -> Write Configuration/Enable
  I2C Master Read/Write/2 -> Bitwise Operator/1

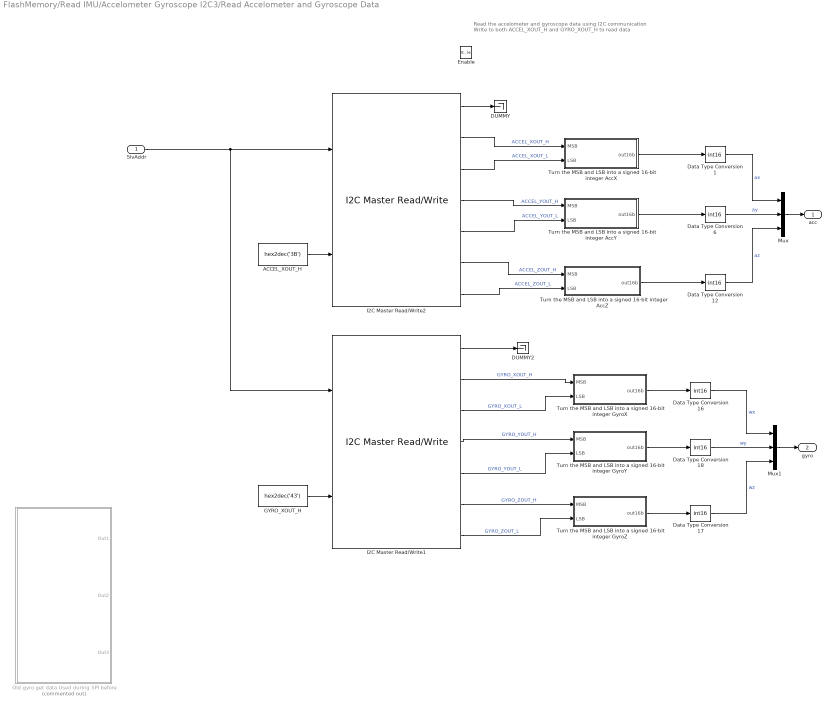
== system FlashMemory/Read IMU/Accelometer Gyroscope I2C3/Read Accelometer and Gyroscope Data ==
  note: Read the accelometer and gyroscope data using I2C communication
      | Write to both ACCEL_XOUT_H and GYRO_XOUT_H to read data
  SlvAddr : Inport
  Enable : EnablePort
  ACCEL_XOUT_H : Constant  Value=hex2dec('3B')  OutDataTypeStr=uint8  SampleTime=-1
  DUMMY : Terminator
  DUMMY2 : Terminator
  Data Type Conversion{1,6,12,16..18} (6 alike) : DataTypeConversion  OutDataTypeStr=int16
  GYRO_XOUT_H : Constant  Value=hex2dec('43')  OutDataTypeStr=uint8  SampleTime=-1
  I2C Master Read/Write1 : stm32f4_i2c_lib/I2C Master Read//Write  configuration=Transaction  module=3  lastmodule=3  transfer=Blocking  dutycycle=TLow/THigh = 2  clkspeed=400  timeout=25  writecount=1  readcount=6  sdapin=C9  sclpin=A8  waitwritetime=0  forcestop=off  inputtypearray=[2 3 3]  outputtypearray=[7 3 3 3 3 3 3 3]  confstr="[\"C\",\"9\",\"A\",\"8\",\"1\",\"3\",\"4\",\"2\",\"I2C_DutyCycle_2\",\"0\",\"off\"]"  sampletime=Ts.IMU  sampletimestr=0.008  blockid=ReadIMUAccelometerGyroscopeI2C3ReadAccelometerandGyroscopeDataI2CMasterReadWrite1
  I2C Master Read/Write2 : stm32f4_i2c_lib/I2C Master Read//Write  configuration=Transaction  module=3  lastmodule=3  transfer=Blocking  dutycycle=TLow/THigh = 2  clkspeed=400  timeout=25  writecount=1  readcount=6  sdapin=C9  sclpin=A8  waitwritetime=0  forcestop=off  inputtypearray=[2 3 3]  outputtypearray=[7 3 3 3 3 3 3 3]  confstr="[\"C\",\"9\",\"A\",\"8\",\"1\",\"3\",\"4\",\"2\",\"I2C_DutyCycle_2\",\"0\",\"off\"]"  sampletime=Ts.IMU  sampletimestr=0.008  blockid=ReadIMUAccelometerGyroscopeI2C3ReadAccelometerandGyroscopeDataI2CMasterReadWrite2
  Mux : Mux  Inputs=3
  Mux1 : Mux  Inputs=3
  Old gyro get data Used during SPI before : Subsystem  Commented=on
  Turn the MSB and LSB into a signed 16-bit integer AccX : Subsystem
  Turn the MSB and LSB into a signed 16-bit integer AccY : Subsystem
  Turn the MSB and LSB into a signed 16-bit integer AccZ : Subsystem
  Turn the MSB and LSB into a signed 16-bit integer GyroX : Subsystem
  Turn the MSB and LSB into a signed 16-bit integer GyroY : Subsystem
  Turn the MSB and LSB into a signed 16-bit integer GyroZ : Subsystem
  acc : Outport
  gyro : Outport  Port=2
  wires:
  I2C Master Read/Write2/1 -> DUMMY/1
  Mux/1 -> acc/1
  Turn the MSB and LSB into a signed 16-bit integer AccX/1(out16b) -> Data Type Conversion1/1
  Turn the MSB and LSB into a signed 16-bit integer AccY/1(out16b) -> Data Type Conversion6/1
  Turn the MSB and LSB into a signed 16-bit integer AccZ/1(out16b) -> Data Type Conversion12/1
  Data Type Conversion1/1 -> Mux/1  "ax"
  Data Type Conversion6/1 -> Mux/2  "ay"
  Data Type Conversion12/1 -> Mux/3  "az"
  I2C Master Read/Write1/1 -> DUMMY2/1
  Mux1/1 -> gyro/1
  Turn the MSB and LSB into a signed 16-bit integer GyroX/1(out16b) -> Data Type Conversion16/1
  Turn the MSB and LSB into a signed 16-bit integer GyroY/1(out16b) -> Data Type Conversion18/1
  Turn the MSB and LSB into a signed 16-bit integer GyroZ/1(out16b) -> Data Type Conversion17/1
  Data Type Conversion16/1 -> Mux1/1  "wx"
  Data Type Conversion18/1 -> Mux1/2  "wy"
  Data Type Conversion17/1 -> Mux1/3  "wz"
  GYRO_XOUT_H/1 -> I2C Master Read/Write1/2
  ACCEL_XOUT_H/1 -> I2C Master Read/Write2/2
  SlvAddr/1 -> I2C Master Read/Write1/1, I2C Master Read/Write2/1
  I2C Master Read/Write2/2 -> Turn the MSB and LSB into a signed 16-bit integer AccX/1(MSB)  "ACCEL_XOUT_H"
  I2C Master Read/Write2/3 -> Turn the MSB and LSB into a signed 16-bit integer AccX/2(LSB)  "ACCEL_XOUT_L"
  I2C Master Read/Write2/5 -> Turn the MSB and LSB into a signed 16-bit integer AccY/2(LSB)  "ACCEL_YOUT_L"
  I2C Master Read/Write2/4 -> Turn the MSB and LSB into a signed 16-bit integer AccY/1(MSB)  "ACCEL_YOUT_H"
  I2C Master Read/Write2/6 -> Turn the MSB and LSB into a signed 16-bit integer AccZ/1(MSB)  "ACCEL_ZOUT_H"
  I2C Master Read/Write2/7 -> Turn the MSB and LSB into a signed 16-bit integer AccZ/2(LSB)  "ACCEL_ZOUT_L"
  I2C Master Read/Write1/2 -> Turn the MSB and LSB into a signed 16-bit integer GyroX/1(MSB)  "GYRO_XOUT_H"
  I2C Master Read/Write1/3 -> Turn the MSB and LSB into a signed 16-bit integer GyroX/2(LSB)  "GYRO_XOUT_L"
  I2C Master Read/Write1/4 -> Turn the MSB and LSB into a signed 16-bit integer GyroY/1(MSB)  "GYRO_YOUT_H"
  I2C Master Read/Write1/5 -> Turn the MSB and LSB into a signed 16-bit integer GyroY/2(LSB)  "GYRO_YOUT_L"
  I2C Master Read/Write1/6 -> Turn the MSB and LSB into a signed 16-bit integer GyroZ/1(MSB)  "GYRO_ZOUT_H"
  I2C Master Read/Write1/7 -> Turn the MSB and LSB into a signed 16-bit integer GyroZ/2(LSB)  "GYRO_ZOUT_L"

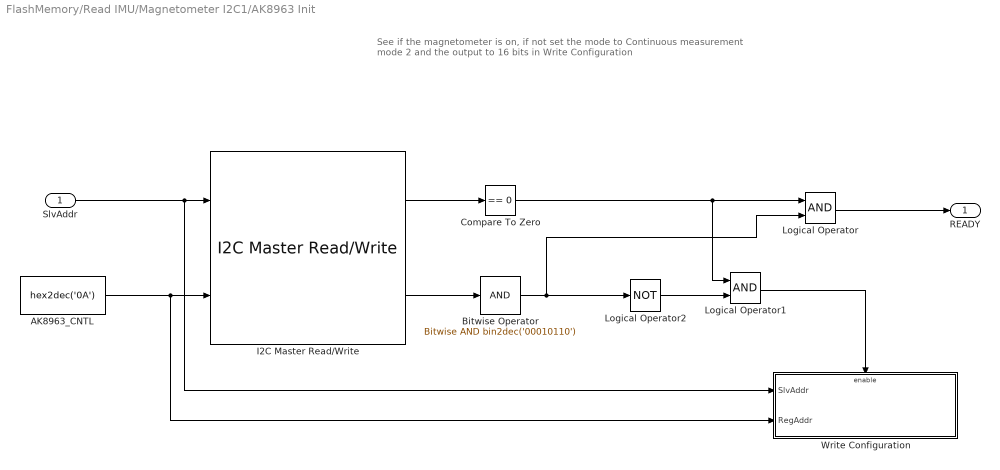
== system FlashMemory/Read IMU/Magnetometer I2C1/AK8963 Init  ==
  note: See if the magnetometer is on, if not
      | set the mode to  Continuous measurement mode 2 and the output to 16 bits
      | in Write Configuration
  SlvAddr : Inport
  AK8963_CNTL : Constant  Value=hex2dec('0A')  OutDataTypeStr=uint8  SampleTime=-1
  Bitwise Operator : simulink/Logic and Bit Operations/Bitwise Operator  logicop=AND  UseBitMask=on  BitMask=bin2dec('00010110')  BitMaskRealWorld=Stored Integer
  Compare To Zero : simulink/Logic and Bit Operations/Compare To Zero  relop===  OutDataTypeStr=boolean
  I2C Master Read/Write : stm32f4_i2c_lib/I2C Master Read//Write  configuration=Transaction  module=1  lastmodule=3  transfer=Blocking  dutycycle=TLow/THigh = 2  clkspeed=400  timeout=25  writecount=1  readcount=1  sdapin=C9  sclpin=A8  waitwritetime=0  forcestop=off  inputtypearray=[2 3 3]  outputtypearray=[2 3 3]  confstr="[\"C\",\"9\",\"A\",\"8\",\"1\",\"1\",\"6\",\"0\",\"I2C_DutyCycle_2\",\"0\",\"off\"]"  sampletime=-1  sampletimestr=0.002  blockid=ReadIMUMagnetometerI2CAK8963InitI2CMasterReadWrite
  Logical Operator : Logic  AllPortsSameDT=off  OutDataTypeStr=boolean
  Logical Operator1 : Logic  AllPortsSameDT=off  OutDataTypeStr=boolean
  Logical Operator2 : Logic  Operator=NOT  AllPortsSameDT=off  OutDataTypeStr=boolean
  Write Configuration : Subsystem
  READY : Outport
  wires:
  SlvAddr/1 -> Write Configuration/1(SlvAddr), I2C Master Read/Write/1
  AK8963_CNTL/1 -> Write Configuration/2(RegAddr), I2C Master Read/Write/2
  I2C Master Read/Write/1 -> Compare To Zero/1
  Logical Operator/1 -> READY/1
  Bitwise Operator/1 -> Logical Operator2/1, Logical Operator/2
  Compare To Zero/1 -> Logical Operator/1, Logical Operator1/1
  I2C Master Read/Write/2 -> Bitwise Operator/1
  Logical Operator2/1 -> Logical Operator1/2
  Logical Operator1/1 -> Write Configuration/Enable

== system FlashMemory/Read IMU/Magnetometer I2C1/Magnetometer Data Ready  ==
  note: Check if magnetometer data is ready
  SlvAddr : Inport
  Enable : EnablePort
  AK8963_ST1 : Constant  Value=hex2dec('02')  OutDataTypeStr=uint8  SampleTime=-1
  Bitwise Operator : simulink/Logic and Bit Operations/Bitwise Operator  logicop=AND  UseBitMask=on  BitMask=bin2dec('00000001')  BitMaskRealWorld=Stored Integer
  Compare To Zero : simulink/Logic and Bit Operations/Compare To Zero  relop===  OutDataTypeStr=boolean
  I2C Master Read/Write : stm32f4_i2c_lib/I2C Master Read//Write  configuration=Transaction  module=1  lastmodule=3  transfer=Blocking  dutycycle=TLow/THigh = 2  clkspeed=400  timeout=25  writecount=1  readcount=1  sdapin=C9  sclpin=A8  waitwritetime=0  forcestop=off  inputtypearray=[2 3 3]  outputtypearray=[2 3 3]  confstr="[\"C\",\"9\",\"A\",\"8\",\"1\",\"1\",\"6\",\"0\",\"I2C_DutyCycle_2\",\"0\",\"off\"]"  sampletime=-1  sampletimestr=0.002  blockid=ReadIMUMagnetometerI2CMagnetometerDataReadyI2CMasterReadWrite
  Logical Operator : Logic  AllPortsSameDT=off  OutDataTypeStr=boolean
  READY : Outport
  wires:
  SlvAddr/1 -> I2C Master Read/Write/1
  AK8963_ST1/1 -> I2C Master Read/Write/2
  I2C Master Read/Write/2 -> Bitwise Operator/1
  I2C Master Read/Write/1 -> Compare To Zero/1
  Compare To Zero/1 -> Logical Operator/1
  Bitwise Operator/1 -> Logical Operator/2
  Logical Operator/1 -> READY/1

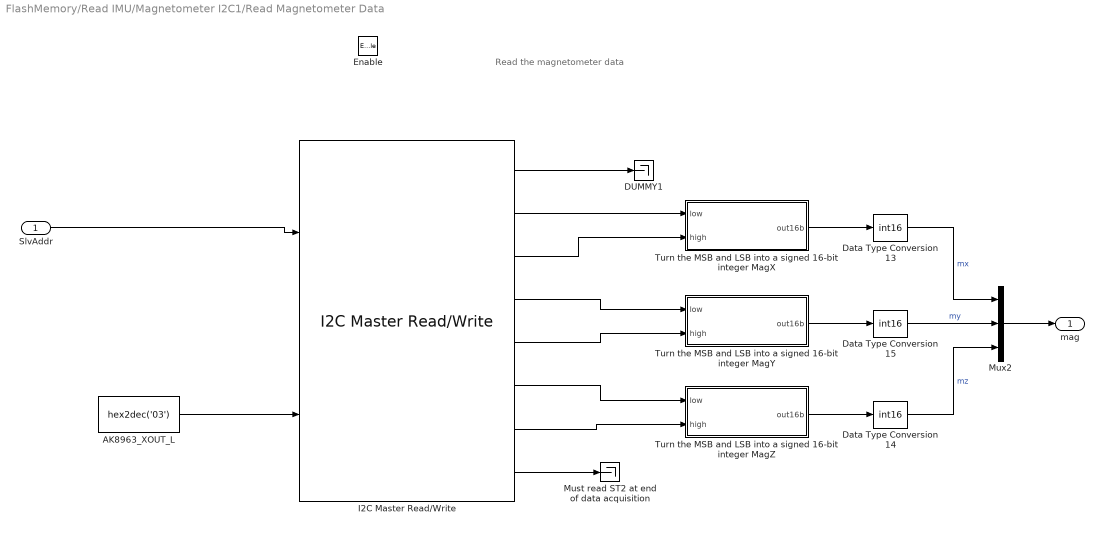
== system FlashMemory/Read IMU/Magnetometer I2C1/Read Magnetometer Data ==
  note: Read the magnetometer data
  "SlvAddr " : Inport
  Enable : EnablePort
  AK8963_XOUT_L : Constant  Value=hex2dec('03')  OutDataTypeStr=uint8  SampleTime=-1
  DUMMY1 : Terminator
  Data Type Conversion13 : DataTypeConversion  OutDataTypeStr=int16
  Data Type Conversion14 : DataTypeConversion  OutDataTypeStr=int16
  Data Type Conversion15 : DataTypeConversion  OutDataTypeStr=int16
  I2C Master Read/Write : stm32f4_i2c_lib/I2C Master Read//Write  configuration=Transaction  module=1  lastmodule=3  transfer=Blocking  dutycycle=TLow/THigh = 2  clkspeed=400  timeout=25  writecount=1  readcount=7  sdapin=C9  sclpin=A8  waitwritetime=0  forcestop=off  inputtypearray=[2 3 3]  outputtypearray=[8 3 3 3 3 3 3 3 3]  confstr="[\"C\",\"9\",\"A\",\"8\",\"1\",\"1\",\"6\",\"0\",\"I2C_DutyCycle_2\",\"0\",\"off\"]"  sampletime=-1  sampletimestr=0.002  blockid=ReadIMUMagnetometerI2CReadMagnetometerDataI2CMasterReadWrite
  "Must read ST2 at end of data acquisition  " : Terminator
  Mux2 : Mux  Inputs=3
  Turn the MSB and LSB into a signed 16-bit integer MagX : Subsystem
  Turn the MSB and LSB into a signed 16-bit integer MagY : Subsystem
  Turn the MSB and LSB into a signed 16-bit integer MagZ : Subsystem
  mag : Outport
  wires:
  Turn the MSB and LSB into a signed 16-bit integer MagX/1(out16b) -> Data Type Conversion13/1
  Turn the MSB and LSB into a signed 16-bit integer MagY/1(out16b) -> Data Type Conversion15/1
  Turn the MSB and LSB into a signed 16-bit integer MagZ/1(out16b) -> Data Type Conversion14/1
  Data Type Conversion13/1 -> Mux2/1  "mx"
  Data Type Conversion15/1 -> Mux2/2  "my"
  Data Type Conversion14/1 -> Mux2/3  "mz"
  AK8963_XOUT_L/1 -> I2C Master Read/Write/2
  I2C Master Read/Write/1 -> DUMMY1/1
  "SlvAddr "/1 -> I2C Master Read/Write/1
  Mux2/1 -> mag/1
  I2C Master Read/Write/8 -> "Must read ST2 at end of data acquisition  "/1
  I2C Master Read/Write/3 -> Turn the MSB and LSB into a signed 16-bit integer MagX/2(high)
  I2C Master Read/Write/2 -> Turn the MSB and LSB into a signed 16-bit integer MagX/1(low)
  I2C Master Read/Write/4 -> Turn the MSB and LSB into a signed 16-bit integer MagY/1(low)
  I2C Master Read/Write/5 -> Turn the MSB and LSB into a signed 16-bit integer MagY/2(high)
  I2C Master Read/Write/6 -> Turn the MSB and LSB into a signed 16-bit integer MagZ/1(low)
  I2C Master Read/Write/7 -> Turn the MSB and LSB into a signed 16-bit integer MagZ/2(high)

== system FlashMemory/Read IMU/SPI3/Turn the MSB and LSB into a signed 16-bit integer AccX ==
  MSB : Inport
  LSB : Inport  Port=2
  Bitwise Operator2 : simulink/Logic and Bit Operations/Bitwise Operator  logicop=OR  UseBitMask=off  NumInputPorts=2  BitMask=bin2dec('11011001')  BitMaskRealWorld=Stored Integer
  Data Type Conversion6 : DataTypeConversion  OutDataTypeStr=uint16
  Data Type Conversion7 : DataTypeConversion  OutDataTypeStr=uint16
  Shift Arithmetic2 : ArithShift  BitShiftNumber=-8
  out16b : Outport
  wires:
  LSB/1 -> Data Type Conversion6/1
  Bitwise Operator2/1 -> out16b/1
  MSB/1 -> Data Type Conversion7/1
  Data Type Conversion7/1 -> Shift Arithmetic2/1
  Data Type Conversion6/1 -> Bitwise Operator2/2
  Shift Arithmetic2/1 -> Bitwise Operator2/1

== system FlashMemory/Read IMU/SPI3/Turn the MSB and LSB into a signed 16-bit integer AccY ==
  MSB : Inport
  LSB : Inport  Port=2
  Bitwise Operator2 : simulink/Logic and Bit Operations/Bitwise Operator  logicop=OR  UseBitMask=off  NumInputPorts=2  BitMask=bin2dec('11011001')  BitMaskRealWorld=Stored Integer
  Data Type Conversion6 : DataTypeConversion  OutDataTypeStr=int16
  Data Type Conversion7 : DataTypeConversion  OutDataTypeStr=int16
  Shift Arithmetic2 : ArithShift  BitShiftNumber=-8
  out16b : Outport
  wires:
  LSB/1 -> Data Type Conversion6/1
  Bitwise Operator2/1 -> out16b/1
  MSB/1 -> Data Type Conversion7/1
  Data Type Conversion7/1 -> Shift Arithmetic2/1
  Data Type Conversion6/1 -> Bitwise Operator2/2
  Shift Arithmetic2/1 -> Bitwise Operator2/1

== system FlashMemory/Read IMU/SPI3/Turn the MSB and LSB into a signed 16-bit integer AccZ ==
  MSB : Inport
  LSB : Inport  Port=2
  Bitwise Operator2 : simulink/Logic and Bit Operations/Bitwise Operator  logicop=OR  UseBitMask=off  NumInputPorts=2  BitMask=bin2dec('11011001')  BitMaskRealWorld=Stored Integer
  Data Type Conversion6 : DataTypeConversion  OutDataTypeStr=int16
  Data Type Conversion7 : DataTypeConversion  OutDataTypeStr=int16
  Shift Arithmetic2 : ArithShift  BitShiftNumber=-8
  out16b : Outport
  wires:
  LSB/1 -> Data Type Conversion6/1
  Bitwise Operator2/1 -> out16b/1
  MSB/1 -> Data Type Conversion7/1
  Data Type Conversion7/1 -> Shift Arithmetic2/1
  Data Type Conversion6/1 -> Bitwise Operator2/2
  Shift Arithmetic2/1 -> Bitwise Operator2/1

== system FlashMemory/Read IMU/SPI3/Turn the MSB and LSB into a signed 16-bit integer GyroX ==
  MSB : Inport
  LSB : Inport  Port=2
  Bitwise Operator2 : simulink/Logic and Bit Operations/Bitwise Operator  logicop=OR  UseBitMask=off  NumInputPorts=2  BitMask=bin2dec('11011001')  BitMaskRealWorld=Stored Integer
  Data Type Conversion1 : DataTypeConversion  OutDataTypeStr=int16
  Data Type Conversion7 : DataTypeConversion  OutDataTypeStr=int16
  Shift Arithmetic2 : ArithShift  BitShiftNumber=-8
  out16b : Outport
  wires:
  MSB/1 -> Data Type Conversion7/1
  Data Type Conversion7/1 -> Shift Arithmetic2/1
  Shift Arithmetic2/1 -> Bitwise Operator2/1
  LSB/1 -> Data Type Conversion1/1
  Data Type Conversion1/1 -> Bitwise Operator2/2
  Bitwise Operator2/1 -> out16b/1

== system FlashMemory/Read IMU/SPI3/Turn the MSB and LSB into a signed 16-bit integer GyroY ==
  MSB : Inport
  LSB : Inport  Port=2
  Bitwise Operator2 : simulink/Logic and Bit Operations/Bitwise Operator  logicop=OR  UseBitMask=off  NumInputPorts=2  BitMask=bin2dec('11011001')  BitMaskRealWorld=Stored Integer
  Data Type Conversion6 : DataTypeConversion  OutDataTypeStr=uint16
  Data Type Conversion7 : DataTypeConversion  OutDataTypeStr=uint16
  Shift Arithmetic2 : ArithShift  BitShiftNumber=-8
  out16b : Outport
  wires:
  LSB/1 -> Data Type Conversion6/1
  Bitwise Operator2/1 -> out16b/1
  MSB/1 -> Data Type Conversion7/1
  Data Type Conversion7/1 -> Shift Arithmetic2/1
  Data Type Conversion6/1 -> Bitwise Operator2/2
  Shift Arithmetic2/1 -> Bitwise Operator2/1
